simulink model "diagram_digital_vector"  (Simulink 7.5)
settings: Solver=ode4  StartTime=0.0  StopTime=10.0  FixedStep=0.001  RelTol=1e-3
PreLoadFcn:
  | diagram_digital_vector_param
values from neighbouring files (symbols this model uses):
  A = [ 0  1  0;       0  0  1;      -6 -3 -2]    [diagram_digital_vector_param.m]
  B = [0;  0;  1]    [diagram_digital_vector_param.m]
  C = [1  0  1]    [diagram_digital_vector_param.m]
  x0 = [0; 0; 0]    [diagram_digital_vector_param.m]
settings Model: Creator=Dell  LastModifiedBy=huiliang

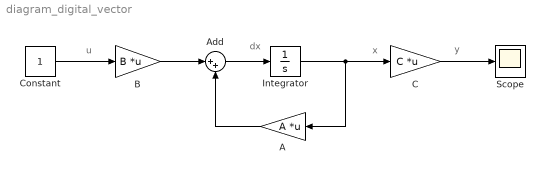
== system diagram_digital_vector ==
  note: x
  note: dx
  note: u
  note: y
  A : Gain  Gain=A  Multiplication=Matrix(K*u)  ParameterDataType=fixdt(1, 16)  ParameterScaling=2^0  OutDataType=fixdt(1, 16)  OutScaling=2^0
  Add : Sum  Inputs=|++  OutDataType=fixdt(1, 16)  OutScaling=2^-10
  B : Gain  Gain=B  Multiplication=Matrix(K*u)  ParameterDataType=fixdt(1, 16)  ParameterScaling=2^0  OutDataType=fixdt(1, 16)  OutScaling=2^0
  C : Gain  Gain=C  Multiplication=Matrix(K*u)  ParameterDataType=fixdt(1, 16)  ParameterScaling=2^0  OutDataType=fixdt(1, 16)  OutScaling=2^0
  Constant : Constant  OutDataType=fixdt(1, 16)  OutScaling=2^0
  Integrator : Integrator  InitialCondition=x0
  Scope : Scope
      settings: TimeRange=10  YMin=-0.2  YMax=0.6000000000000001  MaxDataPoints=10000
  wires:
  Integrator/1 -> A/1, C/1
  Add/1 -> Integrator/1
  A/1 -> Add/2
  B/1 -> Add/1
  Constant/1 -> B/1
  C/1 -> Scope/1
